simulink model "DSR_sim"  (R2021a)
settings: Solver=VariableStepAuto  StartTime=0.0  StopTime=15  RelTol=1e-3
undefined symbols (not defined in the file or in its folder): a, alpha, betac, delay, delay_a, omega
(part 1 of 2)
settings Model: Creator=shiva  LastModifiedBy=shiva

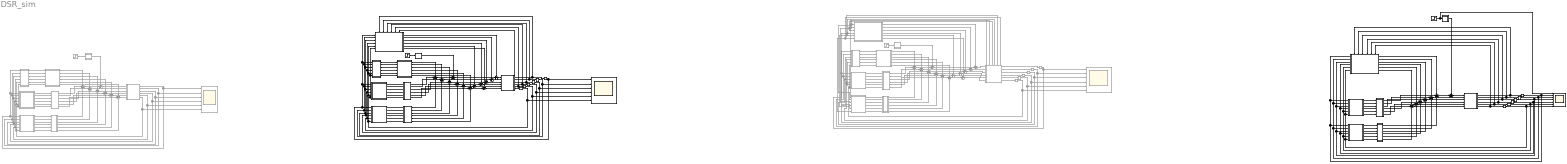
== system DSR_sim ==
  note: Standard Consensus
  note: DSR with velocity derivative
  note: System with accessible velocities
  ConsSys : Subsystem
  Damping : Subsystem
      settings: PortSchema="{\"entries\":[{\"content\":{\"sides\":[{\"content\":{\"connectorIds\":[\"In1\",\"In2\",\"In3\",\"In4\",\"In5\",\"In6\"]},\"type\":\"ConnectorPlacement.EquallySpacedRectSide\",\"uuid\":\"b372a7be-6970-4f0c-9c0a-91cfb5e8dee7\"},{\"content\":{\"connectorIds\":[\"Out1\",\"Out2\",\"Out3\",\"Out4\",\"Out5\",\"Out6\"],\"side\":\"RIGHT\"},\"type\":\"ConnectorPlacement.EquallySpacedRectSide\",\"uuid\":\"0b2444b3-7469-468f-9337-a7c17c408c74\"},{\"content\":{\"connectorIds\":[\"In7\",\"In8\",\"In9\",\"In10\",\"In11\",\"In12\"],\"side\":\"TOP\"},\"type\":\"ConnectorPlacement.EquallySpacedRectSide\",\"uuid\":\"794abe9b-397a-493b-b826-dc3a29ebdba9\"}]},\"type\":\"ConnectorPlacement.EquallySpacedConnector\",\"uuid\":\"dc72dcb4-42f7-41e7-aada-30e307c7b164\"}],\"packageUris\":[\"http://schema.mathworks.com/mf0/Connector/R2020b\"],\"version\":\"1.0\"}"
  Damping1 : Subsystem  Commented=on
  Damping2 : Subsystem
      settings: PortSchema="{\"entries\":[{\"content\":{\"sides\":[{\"content\":{\"connectorIds\":[\"In1\",\"In2\",\"In3\",\"In4\",\"In5\",\"In6\"]},\"type\":\"ConnectorPlacement.EquallySpacedRectSide\",\"uuid\":\"b372a7be-6970-4f0c-9c0a-91cfb5e8dee7\"},{\"content\":{\"connectorIds\":[\"Out1\",\"Out2\",\"Out3\",\"Out4\",\"Out5\",\"Out6\"],\"side\":\"RIGHT\"},\"type\":\"ConnectorPlacement.EquallySpacedRectSide\",\"uuid\":\"0b2444b3-7469-468f-9337-a7c17c408c74\"},{\"content\":{\"connectorIds\":[\"In7\",\"In8\",\"In9\",\"In10\",\"In11\",\"In12\"],\"side\":\"TOP\"},\"type\":\"ConnectorPlacement.EquallySpacedRectSide\",\"uuid\":\"794abe9b-397a-493b-b826-dc3a29ebdba9\"}]},\"type\":\"ConnectorPlacement.EquallySpacedConnector\",\"uuid\":\"dc72dcb4-42f7-41e7-aada-30e307c7b164\"}],\"packageUris\":[\"http://schema.mathworks.com/mf0/Connector/R2020b\"],\"version\":\"1.0\"}"
  DerEst : Subsystem  Commented=on
  DerEst1 : Subsystem
  DerEst2 : Subsystem  Commented=on
  I-beta*K : Subsystem  Commented=on
  I-beta*K1 : Subsystem
  I-beta*K2 : Subsystem  Commented=on
  Input Processor : Subsystem  Commented=on
  Input Processor1 : Subsystem
  Input Processor2 : Subsystem  Commented=on
  Input Processor3 : Subsystem
  KDgain : Subsystem  Commented=on
  KDgain1 : Subsystem
  KDgain2 : Subsystem  Commented=on
  KDgain3 : Subsystem
  KPgain : Subsystem  Commented=on
  KPgain1 : Subsystem
  KPgain2 : Subsystem  Commented=on
  KPgain3 : Subsystem
  KX : Subsystem  Commented=on
  KX1 : Subsystem
  KX2 : Subsystem  Commented=on
  KX3 : Subsystem
  KX_dot : Subsystem  Commented=on
  KX_dot1 : Subsystem
  KX_dot2 : Subsystem  Commented=on
  KX_dot3 : Subsystem
  Scope : Scope  Commented=on  NumInputPorts=6
  Scope1 : Scope  NumInputPorts=6
  Scope2 : Scope  Commented=on  NumInputPorts=6
  Scope4 : Scope  NumInputPorts=7
  Step : Step  Commented=on  SampleTime=0
  Step1 : Step  Time=0  SampleTime=0
  Step2 : Step  Commented=on  Time=0  SampleTime=0
  Step4 : Step  Time=0  SampleTime=0
  Sum{,1..5,20..22,30..32} (12 alike) : Sum  Commented=on  Inputs=+--
  Sum{7..12} (6 alike) : Sum  Inputs=+--
  Sum13 : Sum  Inputs=++|
  Sum{14..19} (6 alike) : Sum  Inputs=-+|
  Sum23 : Sum  Commented=on  Inputs=++|
  Sum{24..29} (6 alike) : Sum  Commented=on  Inputs=-+|
  Sum44 : Sum  Inputs=++|
  Sum{45..50} (6 alike) : Sum  Inputs=---
  Sum6 : Sum  Commented=on  Inputs=++|
  Transport Delay{,1..5,12..17} (12 alike) : TransportDelay  DelayTime=delay_a
  Transport Delay{6..11} (6 alike) : TransportDelay  Commented=on  DelayTime=delay_a
  system : Subsystem  Commented=on
  system1 : Subsystem
  system2 : Subsystem  Commented=on
      settings: PortSchema="{\"entries\":[{\"content\":{\"sides\":[{\"content\":{\"connectorIds\":[\"In1\",\"In2\",\"In3\",\"In4\",\"In5\",\"In6\"]},\"type\":\"ConnectorPlacement.EquallySpacedRectSide\",\"uuid\":\"0544da1f-0f67-4d19-801a-c3e0761d5fdd\"},{\"content\":{\"connectorIds\":[\"Out1\",\"Out2\",\"Out3\",\"Out4\",\"Out5\",\"Out6\"],\"side\":\"RIGHT\"},\"type\":\"ConnectorPlacement.EquallySpacedRectSide\",\"uuid\":\"07850a4a-c00e-49e5-b307-7878de70a2bd\"},{\"content\":{\"connectorIds\":[\"Out7\",\"Out8\",\"Out9\",\"Out10\",\"Out11\",\"Out12\"],\"side\":\"TOP\"},\"type\":\"ConnectorPlacement.EquallySpacedRectSide\",\"uuid\":\"1abf911a-7163-4aef-a115-7988dbad9a54\"}]},\"type\":\"ConnectorPlacement.EquallySpacedConnector\",\"uuid\":\"835a7fab-0379-4bf8-b1b3-ead7ebcc18b2\"}],\"packageUris\":[\"http://schema.mathworks.com/mf0/Connector/R2020b\"],\"version\":\"1.0\"}"
  wires:
  DerEst/1(est) -> I-beta*K/1(Input)
  DerEst/2(est1) -> I-beta*K/2(Input1)
  DerEst/3(est2) -> I-beta*K/3(Input2)
  DerEst/4(est3) -> I-beta*K/4(Input3)
  DerEst/5(est4) -> I-beta*K/5(Input4)
  DerEst/6(est5) -> I-beta*K/6(Input5)
  KX/1(Output) -> KPgain/1(Output)
  KX/2(Output1) -> KPgain/2(Output1)
  KX/3(Output2) -> KPgain/3(Output2)
  KX/4(Output3) -> KPgain/4(Output3)
  KX/5(Output4) -> KPgain/5(Output4)
  KX/6(Output5) -> KPgain/6(Output5)
  KX_dot/1(Output) -> KDgain/1(Output)
  KX_dot/2(Output1) -> KDgain/2(Output1)
  KX_dot/3(Output2) -> KDgain/3(Output2)
  KX_dot/4(Output3) -> KDgain/4(Output3)
  KX_dot/5(Output4) -> KDgain/5(Output4)
  KX_dot/6(Output5) -> KDgain/6(Output5)
  system/1(Ag1) -> KX_dot/1(Input), KX/1(Input), DerEst/1(pos), Scope/1
  system/2(Ag2) -> KX_dot/2(Input1), KX/2(Input1), DerEst/2(pos1), Scope/2
  system/3(Ag3) -> KX_dot/3(Input2), KX/3(Input2), DerEst/3(pos2), Scope/3
  system/4(Ag4) -> KX_dot/4(Input3), KX/4(Input3), DerEst/4(pos3), Scope/4
  system/5(Ag5) -> KX_dot/5(Input4), KX/5(Input4), DerEst/5(pos4), Scope/5
  system/6(Ag6) -> DerEst/6(pos5), KX/6(Input5), KX_dot/6(Input5), Scope/6
  Sum1/1 -> system/2(In2)
  Sum5/1 -> system/6(In6)
  Sum4/1 -> system/5(In5)
  Sum3/1 -> system/4(In4)
  Sum2/1 -> system/3(In3)
  Step/1 -> Input Processor/1(Input)
  Sum/1 -> Sum6/2
  Sum6/1 -> system/1(In1)
  Input Processor/1(Out1) -> Sum6/1
  I-beta*K/1(Output) -> Sum/1
  KPgain/1(Out1) -> Sum/2
  KDgain/1(Out1) -> Sum/3
  I-beta*K/2(Output1) -> Sum1/1
  KPgain/2(Out2) -> Sum1/2
  KDgain/2(Out2) -> Sum1/3
  I-beta*K/3(Output2) -> Sum2/1
  KPgain/3(Out3) -> Sum2/2
  KDgain/3(Out3) -> Sum2/3
  I-beta*K/4(Output3) -> Sum3/1
  KPgain/4(Out4) -> Sum3/2
  KDgain/4(Out4) -> Sum3/3
  I-beta*K/5(Output4) -> Sum4/1
  KPgain/5(Out5) -> Sum4/2
  KDgain/5(Out5) -> Sum4/3
  I-beta*K/6(Output5) -> Sum5/1
  KPgain/6(Out6) -> Sum5/2
  KDgain/6(Out6) -> Sum5/3
  KX1/4(Output3) -> KPgain1/4(Output3)
  KX1/6(Output5) -> KPgain1/6(Output5)
  KX1/2(Output1) -> KPgain1/2(Output1)
  I-beta*K1/1(Output) -> Sum7/1
  KX_dot1/3(Output2) -> KDgain1/3(Output2)
  I-beta*K1/6(Output5) -> Sum12/1
  system1/5(Ag5) -> Damping/11(Input7), Transport Delay4/1
  system1/4(Ag4) -> Transport Delay3/1, Damping/10(Input8)
  KPgain1/4(Out4) -> Sum10/2
  system1/2(Ag2) -> Transport Delay1/1, Damping/8(Input10)
  I-beta*K1/5(Output4) -> Sum11/1
  KPgain1/3(Out3) -> Sum9/2
  KX1/1(Output) -> KPgain1/1(Output)
  KX_dot1/5(Output4) -> KDgain1/5(Output4)
  system1/3(Ag3) -> Transport Delay2/1, Damping/9(Input9)
  KX_dot1/2(Output1) -> KDgain1/2(Output1)
  KX_dot1/6(Output5) -> KDgain1/6(Output5)
  Step1/1 -> Input Processor1/1(Input)
  KDgain1/4(Out4) -> Sum10/3
  KX1/5(Output4) -> KPgain1/5(Output4)
  KX_dot1/1(Output) -> KDgain1/1(Output)
  I-beta*K1/3(Output2) -> Sum9/1
  KPgain1/1(Out1) -> Sum7/2
  KDgain1/1(Out1) -> Sum7/3
  KDgain1/5(Out5) -> Sum11/3
  system1/6(Ag6) -> Transport Delay5/1, Damping/12(Input6)
  DerEst1/5(est4) -> I-beta*K1/5(Input4)
  system1/1(Ag1) -> Transport Delay/1, Damping/7(Input11)
  KPgain1/6(Out6) -> Sum12/2
  Sum7/1 -> Sum13/2
  I-beta*K1/4(Output3) -> Sum10/1
  KDgain1/3(Out3) -> Sum9/3
  KX1/3(Output2) -> KPgain1/3(Output2)
  Input Processor1/1(Out1) -> Sum13/1
  DerEst1/6(est5) -> I-beta*K1/6(Input5)
  KX_dot1/4(Output3) -> KDgain1/4(Output3)
  DerEst1/2(est1) -> I-beta*K1/2(Input1)
  KPgain1/5(Out5) -> Sum11/2
  KPgain1/2(Out2) -> Sum8/2
  KDgain1/2(Out2) -> Sum8/3
  DerEst1/4(est3) -> I-beta*K1/4(Input3)
  DerEst1/1(est) -> I-beta*K1/1(Input)
  KDgain1/6(Out6) -> Sum12/3
  DerEst1/3(est2) -> I-beta*K1/3(Input2)
  I-beta*K1/2(Output1) -> Sum8/1
  Sum14/1 -> system1/1(In1)
  Sum15/1 -> system1/2(In2)
  Sum16/1 -> system1/3(In3)
  Sum17/1 -> system1/4(In4)
  Sum18/1 -> system1/5(In5)
  Sum19/1 -> system1/6(In6)
  Sum12/1 -> Sum19/2
  Sum11/1 -> Sum18/2
  Sum10/1 -> Sum17/2
  Sum9/1 -> Sum16/2
  Sum8/1 -> Sum15/2
  Sum13/1 -> Sum14/2
  Transport Delay/1 -> KX_dot1/1(Input), KX1/1(Input), DerEst1/1(pos), Damping/1(Input), Scope1/1
  Transport Delay1/1 -> KX_dot1/2(Input1), KX1/2(Input1), DerEst1/2(pos1), Damping/2(Input1), Scope1/2
  Transport Delay2/1 -> KX_dot1/3(Input2), KX1/3(Input2), DerEst1/3(pos2), Damping/3(Input2), Scope1/3
  Transport Delay3/1 -> KX_dot1/4(Input3), KX1/4(Input3), DerEst1/4(pos3), Damping/4(Input3), Scope1/4
  Transport Delay4/1 -> KX_dot1/5(Input4), KX1/5(Input4), DerEst1/5(pos4), Damping/5(Input4), Scope1/5
  Transport Delay5/1 -> Damping/6(Input5), DerEst1/6(pos5), KX1/6(Input5), KX_dot1/6(Input5), Scope1/6
  Damping/1(Out1) -> Sum14/1
  Damping/2(Out2) -> Sum15/1
  Damping/3(Out3) -> Sum16/1
  Damping/4(Out4) -> Sum17/1
  Damping/5(Out5) -> Sum18/1
  Damping/6(Out6) -> Sum19/1
  Damping1/2(Out2) -> Sum25/1
  Damping1/1(Out1) -> Sum24/1
  Damping1/4(Out4) -> Sum27/1
  Damping1/5(Out5) -> Sum28/1
  Transport Delay11/1 -> DerEst2/6(pos5), KX2/6(Input5), Scope2/6
  Sum31/1 -> Sum25/2
  Sum23/1 -> Sum24/2
  Sum22/1 -> Sum29/2
  Sum26/1 -> system2/3(In3)
  Transport Delay10/1 -> KX2/5(Input4), DerEst2/5(pos4), Scope2/5
  Sum28/1 -> system2/5(In5)
  Sum27/1 -> system2/4(In4)
  Sum29/1 -> system2/6(In6)
  Sum20/1 -> Sum27/2
  Sum25/1 -> system2/2(In2)
  KDgain2/5(Out5) -> Sum21/3
  KDgain2/1(Out1) -> Sum30/3
  KPgain2/1(Out1) -> Sum30/2
  KDgain2/4(Out4) -> Sum20/3
  Step2/1 -> Input Processor2/1(Input)
  KX_dot2/1(Output) -> KDgain2/1(Output)
  KX_dot2/6(Output5) -> KDgain2/6(Output5)
  I-beta*K2/3(Output2) -> Sum32/1
  KX2/5(Output4) -> KPgain2/5(Output4)
  system2/3(Ag3) -> Transport Delay8/1
  KX_dot2/2(Output1) -> KDgain2/2(Output1)
  KPgain2/3(Out3) -> Sum32/2
  KX2/1(Output) -> KPgain2/1(Output)
  KX_dot2/5(Output4) -> KDgain2/5(Output4)
  I-beta*K2/5(Output4) -> Sum21/1
  system2/2(Ag2) -> Transport Delay7/1
  KPgain2/4(Out4) -> Sum20/2
  I-beta*K2/6(Output5) -> Sum22/1
  KX2/2(Output1) -> KPgain2/2(Output1)
  KX2/6(Output5) -> KPgain2/6(Output5)
  KPgain2/2(Out2) -> Sum31/2
  KDgain2/2(Out2) -> Sum31/3
  system2/5(Ag5) -> Transport Delay10/1
  DerEst2/1(est) -> I-beta*K2/1(Input)
  DerEst2/2(est1) -> I-beta*K2/2(Input1)
  system2/4(Ag4) -> Transport Delay9/1
  Input Processor2/1(Out1) -> Sum23/1
  KX_dot2/4(Output3) -> KDgain2/4(Output3)
  KX2/3(Output2) -> KPgain2/3(Output2)
  DerEst2/6(est5) -> I-beta*K2/6(Input5)
  Sum32/1 -> Sum26/2
  I-beta*K2/4(Output3) -> Sum20/1
  Sum30/1 -> Sum23/2
  KDgain2/6(Out6) -> Sum22/3
  DerEst2/4(est3) -> I-beta*K2/4(Input3)
  KX_dot2/3(Output2) -> KDgain2/3(Output2)
  KDgain2/3(Out3) -> Sum32/3
  system2/1(Ag1) -> Transport Delay6/1
  KPgain2/6(Out6) -> Sum22/2
  Sum21/1 -> Sum28/2
  DerEst2/5(est4) -> I-beta*K2/5(Input4)
  DerEst2/3(est2) -> I-beta*K2/3(Input2)
  system2/6(Ag6) -> Transport Delay11/1
  Transport Delay9/1 -> KX2/4(Input3), DerEst2/4(pos3), Scope2/4
  Damping1/6(Out6) -> Sum29/1
  Transport Delay6/1 -> KX2/1(Input), DerEst2/1(pos), Scope2/1
  KX2/4(Output3) -> KPgain2/4(Output3)
  I-beta*K2/1(Output) -> Sum30/1
  Transport Delay8/1 -> KX2/3(Input2), DerEst2/3(pos2), Scope2/3
  Transport Delay7/1 -> KX2/2(Input1), DerEst2/2(pos1), Scope2/2
  I-beta*K2/2(Output1) -> Sum31/1
  KPgain2/5(Out5) -> Sum21/2
  Sum24/1 -> system2/1(In1)
  Damping1/3(Out3) -> Sum26/1
  system2/7(Ag7) -> KX_dot2/1(Input), Damping1/1(Input)
  system2/8(Ag8) -> KX_dot2/2(Input1), Damping1/2(Input1)
  system2/9(Ag9) -> KX_dot2/3(Input2), Damping1/3(Input2)
  system2/10(Ag10) -> Damping1/4(Input3), KX_dot2/4(Input3)
  system2/11(Ag11) -> KX_dot2/5(Input4), Damping1/5(Input4)
  system2/12(Ag12) -> Damping1/6(Input5), KX_dot2/6(Input5)
  ConsSys/6(Ag6) -> Damping2/12(Input6), Transport Delay17/1
  ConsSys/5(Ag5) -> Damping2/11(Input7), Transport Delay16/1
  ConsSys/4(Ag4) -> Damping2/10(Input8), Transport Delay15/1
  ConsSys/3(Ag3) -> Damping2/9(Input9), Transport Delay14/1
  ConsSys/2(Ag2) -> Transport Delay13/1, Damping2/8(Input10)
  ConsSys/1(Ag1) -> Damping2/7(Input11), Transport Delay12/1
  KX3/1(Output) -> KPgain3/1(Output)
  KX3/2(Output1) -> KPgain3/2(Output1)
  KX3/3(Output2) -> KPgain3/3(Output2)
  KX3/4(Output3) -> KPgain3/4(Output3)
  KX3/5(Output4) -> KPgain3/5(Output4)
  KX3/6(Output5) -> KPgain3/6(Output5)
  Step4/1 -> Scope4/1, Input Processor3/1(Input)
  KX_dot3/1(Output) -> KDgain3/1(Output)
  KX_dot3/2(Output1) -> KDgain3/2(Output1)
  KX_dot3/3(Output2) -> KDgain3/3(Output2)
  KX_dot3/4(Output3) -> KDgain3/4(Output3)
  KX_dot3/5(Output4) -> KDgain3/5(Output4)
  KX_dot3/6(Output5) -> KDgain3/6(Output5)
  Transport Delay12/1 -> Damping2/1(Input), KX3/1(Input), KX_dot3/1(Input), Scope4/2
  Transport Delay13/1 -> Damping2/2(Input1), KX3/2(Input1), KX_dot3/2(Input1), Scope4/3
  Transport Delay14/1 -> Damping2/3(Input2), KX3/3(Input2), KX_dot3/3(Input2), Scope4/4
  Transport Delay15/1 -> Damping2/4(Input3), KX3/4(Input3), KX_dot3/4(Input3), Scope4/5
  Transport Delay16/1 -> Damping2/5(Input4), KX3/5(Input4), KX_dot3/5(Input4), Scope4/6
  Transport Delay17/1 -> Damping2/6(Input5), KX3/6(Input5), KX_dot3/6(Input5), Scope4/7
  Sum46/1 -> ConsSys/2(In2)
  Sum44/1 -> ConsSys/1(In1)
  Sum45/1 -> Sum44/2
  Sum48/1 -> ConsSys/4(In4)
  Sum49/1 -> ConsSys/5(In5)
  Sum50/1 -> ConsSys/6(In6)
  Sum47/1 -> ConsSys/3(In3)
  Input Processor3/1(Out1) -> Sum44/1
  KPgain3/1(Out1) -> Sum45/2
  KPgain3/2(Out2) -> Sum46/2
  KPgain3/3(Out3) -> Sum47/2
  KPgain3/4(Out4) -> Sum48/2
  KPgain3/5(Out5) -> Sum49/2
  KPgain3/6(Out6) -> Sum50/2
  KDgain3/1(Out1) -> Sum45/3
  KDgain3/2(Out2) -> Sum46/3
  KDgain3/3(Out3) -> Sum47/3
  KDgain3/4(Out4) -> Sum48/3
  KDgain3/5(Out5) -> Sum49/3
  KDgain3/6(Out6) -> Sum50/3
  Damping2/1(Out1) -> Sum45/1
  Damping2/2(Out2) -> Sum46/1
  Damping2/3(Out3) -> Sum47/1
  Damping2/4(Out4) -> Sum48/1
  Damping2/5(Out5) -> Sum49/1
  Damping2/6(Out6) -> Sum50/1

== system DSR_sim/ConsSys ==
  In1 : Inport
  In2 : Inport  Port=2
  In3 : Inport  Port=3
  In4 : Inport  Port=4
  In5 : Inport  Port=5
  In6 : Inport  Port=6
  Transfer Fcn{,1..5} (6 alike) : TransferFcn  Denominator=[1 0 0]
  Ag1 : Outport
  Ag2 : Outport  Port=2
  Ag3 : Outport  Port=3
  Ag4 : Outport  Port=4
  Ag5 : Outport  Port=5
  Ag6 : Outport  Port=6
  wires:
  Transfer Fcn4/1 -> Ag5/1
  In1/1 -> Transfer Fcn/1
  Transfer Fcn/1 -> Ag1/1
  In3/1 -> Transfer Fcn2/1
  Transfer Fcn2/1 -> Ag3/1
  In2/1 -> Transfer Fcn1/1
  In5/1 -> Transfer Fcn4/1
  Transfer Fcn1/1 -> Ag2/1
  In6/1 -> Transfer Fcn5/1
  In4/1 -> Transfer Fcn3/1
  Transfer Fcn5/1 -> Ag6/1
  Transfer Fcn3/1 -> Ag4/1

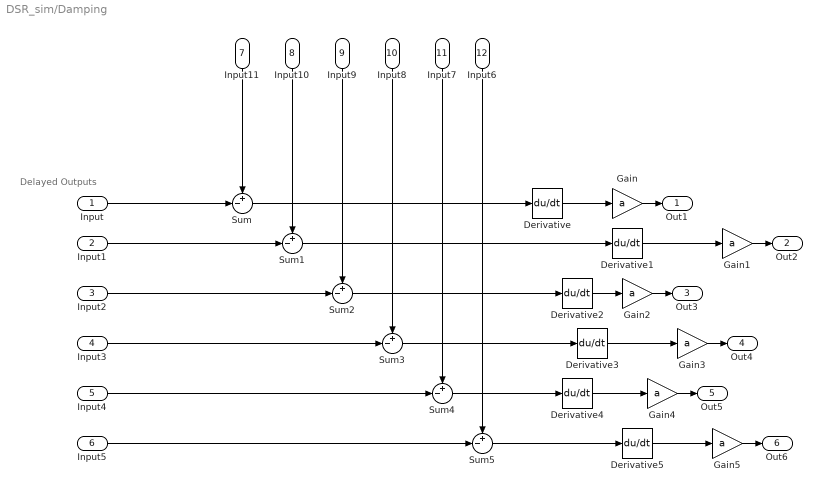
== system DSR_sim/Damping ==
  note: Delayed Outputs
  Input : Inport
  Input1 : Inport  Port=2
  Input2 : Inport  Port=3
  Input3 : Inport  Port=4
  Input4 : Inport  Port=5
  Input5 : Inport  Port=6
  Input11 : Inport  Port=7
  Input10 : Inport  Port=8
  Input9 : Inport  Port=9
  Input8 : Inport  Port=10
  Input7 : Inport  Port=11
  Input6 : Inport  Port=12
  Derivative{,1..5} (6 alike) : Derivative
  Gain{,1..5} (6 alike) : Gain  Gain=a
  Sum{,1..5} (6 alike) : Sum  Inputs=+-|
  Out1 : Outport
  Out2 : Outport  Port=2
  Out3 : Outport  Port=3
  Out4 : Outport  Port=4
  Out5 : Outport  Port=5
  Out6 : Outport  Port=6
  wires:
  Gain5/1 -> Out6/1
  Gain/1 -> Out1/1
  Gain2/1 -> Out3/1
  Gain4/1 -> Out5/1
  Gain3/1 -> Out4/1
  Gain1/1 -> Out2/1
  Input/1 -> Sum/2
  Input11/1 -> Sum/1
  Sum/1 -> Derivative/1
  Input1/1 -> Sum1/2
  Input10/1 -> Sum1/1
  Input2/1 -> Sum2/2
  Input9/1 -> Sum2/1
  Input8/1 -> Sum3/1
  Input3/1 -> Sum3/2
  Input4/1 -> Sum4/2
  Input7/1 -> Sum4/1
  Input5/1 -> Sum5/2
  Input6/1 -> Sum5/1
  Sum1/1 -> Derivative1/1
  Sum2/1 -> Derivative2/1
  Sum3/1 -> Derivative3/1
  Sum4/1 -> Derivative4/1
  Sum5/1 -> Derivative5/1
  Derivative/1 -> Gain/1
  Derivative1/1 -> Gain1/1
  Derivative2/1 -> Gain2/1
  Derivative3/1 -> Gain3/1
  Derivative4/1 -> Gain4/1
  Derivative5/1 -> Gain5/1

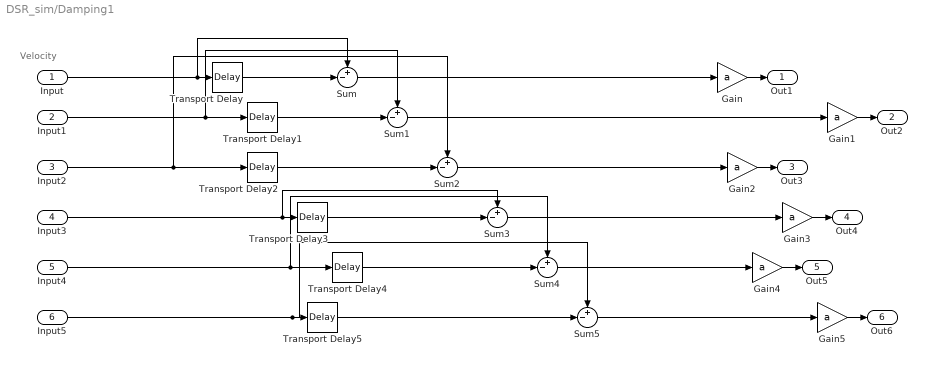
== system DSR_sim/Damping1 ==
  note: Velocity
  Input : Inport
  Input1 : Inport  Port=2
  Input2 : Inport  Port=3
  Input3 : Inport  Port=4
  Input4 : Inport  Port=5
  Input5 : Inport  Port=6
  Gain{,1..5} (6 alike) : Gain  Gain=a
  Sum{,1..5} (6 alike) : Sum  Inputs=+-|
  Transport Delay{,1..5} (6 alike) : TransportDelay  DelayTime=delay_a
  Out1 : Outport
  Out2 : Outport  Port=2
  Out3 : Outport  Port=3
  Out4 : Outport  Port=4
  Out5 : Outport  Port=5
  Out6 : Outport  Port=6
  wires:
  Gain5/1 -> Out6/1
  Gain/1 -> Out1/1
  Gain2/1 -> Out3/1
  Gain4/1 -> Out5/1
  Gain3/1 -> Out4/1
  Gain1/1 -> Out2/1
  Input/1 -> Sum/1, Transport Delay/1
  Input1/1 -> Transport Delay1/1, Sum1/1
  Input2/1 -> Transport Delay2/1, Sum2/1
  Input3/1 -> Sum3/1, Transport Delay3/1
  Input4/1 -> Transport Delay4/1, Sum4/1
  Input5/1 -> Sum5/1, Transport Delay5/1
  Sum/1 -> Gain/1
  Sum1/1 -> Gain1/1
  Sum2/1 -> Gain2/1
  Sum3/1 -> Gain3/1
  Sum4/1 -> Gain4/1
  Sum5/1 -> Gain5/1
  Transport Delay/1 -> Sum/2
  Transport Delay1/1 -> Sum1/2
  Transport Delay2/1 -> Sum2/2
  Transport Delay3/1 -> Sum3/2
  Transport Delay4/1 -> Sum4/2
  Transport Delay5/1 -> Sum5/2

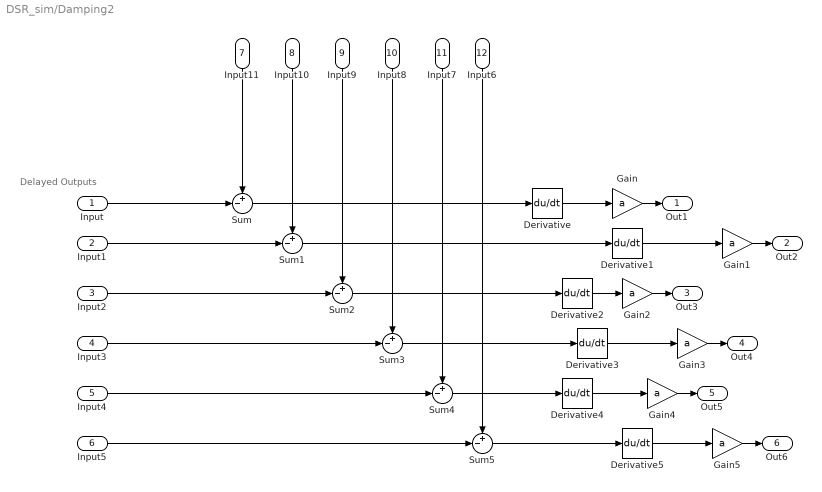
== system DSR_sim/Damping2 ==
  note: Delayed Outputs
  Input : Inport
  Input1 : Inport  Port=2
  Input2 : Inport  Port=3
  Input3 : Inport  Port=4
  Input4 : Inport  Port=5
  Input5 : Inport  Port=6
  Input11 : Inport  Port=7
  Input10 : Inport  Port=8
  Input9 : Inport  Port=9
  Input8 : Inport  Port=10
  Input7 : Inport  Port=11
  Input6 : Inport  Port=12
  Derivative{,1..5} (6 alike) : Derivative
  Gain{,1..5} (6 alike) : Gain  Gain=a
  Sum{,1..5} (6 alike) : Sum  Inputs=+-|
  Out1 : Outport
  Out2 : Outport  Port=2
  Out3 : Outport  Port=3
  Out4 : Outport  Port=4
  Out5 : Outport  Port=5
  Out6 : Outport  Port=6
  wires:
  Gain5/1 -> Out6/1
  Gain/1 -> Out1/1
  Gain2/1 -> Out3/1
  Gain4/1 -> Out5/1
  Gain3/1 -> Out4/1
  Gain1/1 -> Out2/1
  Input/1 -> Sum/2
  Input11/1 -> Sum/1
  Sum/1 -> Derivative/1
  Input1/1 -> Sum1/2
  Input10/1 -> Sum1/1
  Input2/1 -> Sum2/2
  Input9/1 -> Sum2/1
  Input8/1 -> Sum3/1
  Input3/1 -> Sum3/2
  Input4/1 -> Sum4/2
  Input7/1 -> Sum4/1
  Input5/1 -> Sum5/2
  Input6/1 -> Sum5/1
  Sum1/1 -> Derivative1/1
  Sum2/1 -> Derivative2/1
  Sum3/1 -> Derivative3/1
  Sum4/1 -> Derivative4/1
  Sum5/1 -> Derivative5/1
  Derivative/1 -> Gain/1
  Derivative1/1 -> Gain1/1
  Derivative2/1 -> Gain2/1
  Derivative3/1 -> Gain3/1
  Derivative4/1 -> Gain4/1
  Derivative5/1 -> Gain5/1

== system DSR_sim/DerEst ==
  pos : Inport
  pos1 : Inport  Port=2
  pos2 : Inport  Port=3
  pos3 : Inport  Port=4
  pos4 : Inport  Port=5
  pos5 : Inport  Port=6
  Derivative Estimator : Subsystem
  Derivative Estimator1 : Subsystem
  Derivative Estimator2 : Subsystem
  Derivative Estimator3 : Subsystem
  Derivative Estimator4 : Subsystem
  Derivative Estimator5 : Subsystem
  est : Outport
  est1 : Outport  Port=2
  est2 : Outport  Port=3
  est3 : Outport  Port=4
  est4 : Outport  Port=5
  est5 : Outport  Port=6
  wires:
  pos3/1 -> Derivative Estimator3/1(pos)
  Derivative Estimator4/1(est) -> est4/1
  Derivative Estimator2/1(est) -> est2/1
  Derivative Estimator3/1(est) -> est3/1
  Derivative Estimator1/1(est) -> est1/1
  pos1/1 -> Derivative Estimator1/1(pos)
  Derivative Estimator5/1(est) -> est5/1
  Derivative Estimator/1(est) -> est/1
  pos/1 -> Derivative Estimator/1(pos)
  pos2/1 -> Derivative Estimator2/1(pos)
  pos5/1 -> Derivative Estimator5/1(pos)
  pos4/1 -> Derivative Estimator4/1(pos)

== system DSR_sim/DerEst1 ==
  pos : Inport
  pos1 : Inport  Port=2
  pos2 : Inport  Port=3
  pos3 : Inport  Port=4
  pos4 : Inport  Port=5
  pos5 : Inport  Port=6
  Derivative Estimator : Subsystem
  Derivative Estimator1 : Subsystem
  Derivative Estimator2 : Subsystem
  Derivative Estimator3 : Subsystem
  Derivative Estimator4 : Subsystem
  Derivative Estimator5 : Subsystem
  est : Outport
  est1 : Outport  Port=2
  est2 : Outport  Port=3
  est3 : Outport  Port=4
  est4 : Outport  Port=5
  est5 : Outport  Port=6
  wires:
  pos3/1 -> Derivative Estimator3/1(pos)
  Derivative Estimator4/1(est) -> est4/1
  Derivative Estimator2/1(est) -> est2/1
  Derivative Estimator3/1(est) -> est3/1
  Derivative Estimator1/1(est) -> est1/1
  pos1/1 -> Derivative Estimator1/1(pos)
  Derivative Estimator5/1(est) -> est5/1
  Derivative Estimator/1(est) -> est/1
  pos/1 -> Derivative Estimator/1(pos)
  pos2/1 -> Derivative Estimator2/1(pos)
  pos5/1 -> Derivative Estimator5/1(pos)
  pos4/1 -> Derivative Estimator4/1(pos)

== system DSR_sim/DerEst2 ==
  pos : Inport
  pos1 : Inport  Port=2
  pos2 : Inport  Port=3
  pos3 : Inport  Port=4
  pos4 : Inport  Port=5
  pos5 : Inport  Port=6
  Derivative Estimator : Subsystem
  Derivative Estimator1 : Subsystem
  Derivative Estimator2 : Subsystem
  Derivative Estimator3 : Subsystem
  Derivative Estimator4 : Subsystem
  Derivative Estimator5 : Subsystem
  est : Outport
  est1 : Outport  Port=2
  est2 : Outport  Port=3
  est3 : Outport  Port=4
  est4 : Outport  Port=5
  est5 : Outport  Port=6
  wires:
  pos3/1 -> Derivative Estimator3/1(pos)
  Derivative Estimator4/1(est) -> est4/1
  Derivative Estimator2/1(est) -> est2/1
  Derivative Estimator3/1(est) -> est3/1
  Derivative Estimator1/1(est) -> est1/1
  pos1/1 -> Derivative Estimator1/1(pos)
  Derivative Estimator5/1(est) -> est5/1
  Derivative Estimator/1(est) -> est/1
  pos/1 -> Derivative Estimator/1(pos)
  pos2/1 -> Derivative Estimator2/1(pos)
  pos5/1 -> Derivative Estimator5/1(pos)
  pos4/1 -> Derivative Estimator4/1(pos)

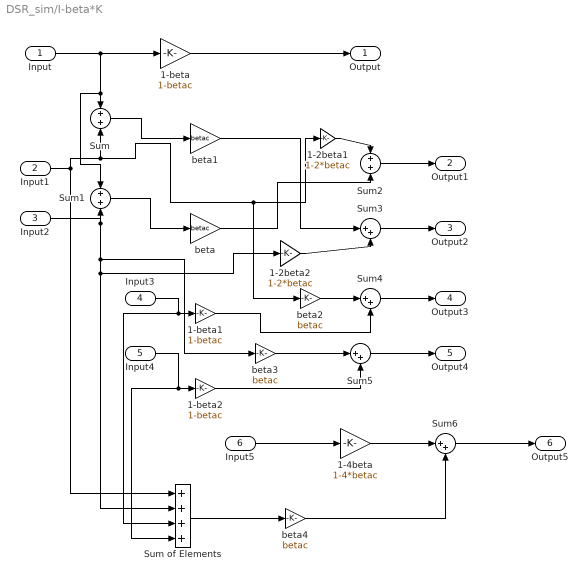
== system DSR_sim/I-beta*K ==
  Input : Inport
  Input1 : Inport  Port=2
  Input2 : Inport  Port=3
  Input3 : Inport  Port=4
  Input4 : Inport  Port=5
  Input5 : Inport  Port=6
  1-2beta1 : Gain  Gain=1-2*betac
  1-2beta2 : Gain  Gain=1-2*betac
  1-4beta : Gain  Gain=1-4*betac
  1-beta : Gain  Gain=1-betac
  1-beta1 : Gain  Gain=1-betac
  1-beta2 : Gain  Gain=1-betac
  Sum : Sum  Inputs=+|+
  Sum of Elements : Sum  Inputs=++++
  Sum1 : Sum  Inputs=+|+
  Sum2 : Sum  Inputs=+|+
  Sum{3..6} (4 alike) : Sum  Inputs=|++
  beta{,1..4} (5 alike) : Gain  Gain=betac
  Output : Outport
  Output1 : Outport  Port=2
  Output2 : Outport  Port=3
  Output3 : Outport  Port=4
  Output4 : Outport  Port=5
  Output5 : Outport  Port=6
  wires:
  Input/1 -> 1-beta/1, Sum1/1, Sum/1
  1-2beta2/1 -> Sum3/2
  1-beta2/1 -> Sum5/2
  Sum4/1 -> Output3/1
  1-beta/1 -> Output/1
  beta/1 -> Sum2/2
  Sum6/1 -> Output5/1
  1-beta1/1 -> Sum4/2
  Input2/1 -> Sum of Elements/2, 1-2beta2/1, beta3/1, Sum1/2
  1-2beta1/1 -> Sum2/1
  Input1/1 -> 1-2beta1/1, beta2/1, Sum/2, Sum of Elements/1
  beta4/1 -> Sum6/2
  Sum/1 -> beta1/1
  Input3/1 -> Sum of Elements/3, 1-beta1/1
  beta3/1 -> Sum5/1
  beta1/1 -> Sum3/1
  beta2/1 -> Sum4/1
  Sum5/1 -> Output4/1
  Input4/1 -> Sum of Elements/4, 1-beta2/1
  Sum1/1 -> beta/1
  1-4beta/1 -> Sum6/1
  Sum2/1 -> Output1/1
  Sum3/1 -> Output2/1
  Input5/1 -> 1-4beta/1
  Sum of Elements/1 -> beta4/1

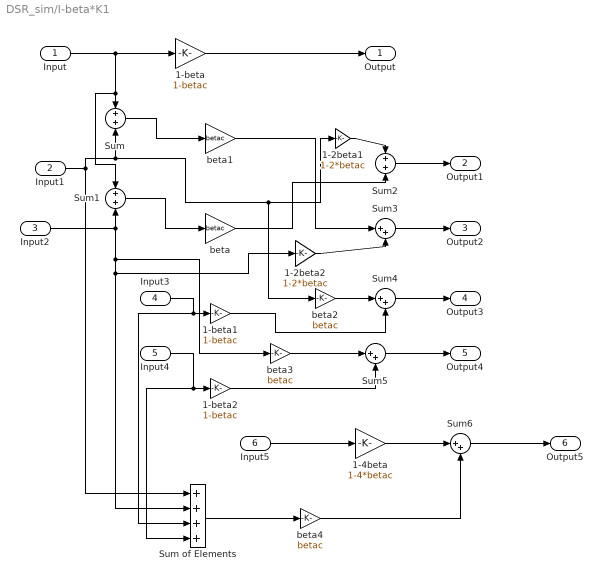
== system DSR_sim/I-beta*K1 ==
  Input : Inport
  Input1 : Inport  Port=2
  Input2 : Inport  Port=3
  Input3 : Inport  Port=4
  Input4 : Inport  Port=5
  Input5 : Inport  Port=6
  1-2beta1 : Gain  Gain=1-2*betac
  1-2beta2 : Gain  Gain=1-2*betac
  1-4beta : Gain  Gain=1-4*betac
  1-beta : Gain  Gain=1-betac
  1-beta1 : Gain  Gain=1-betac
  1-beta2 : Gain  Gain=1-betac
  Sum : Sum  Inputs=+|+
  Sum of Elements : Sum  Inputs=++++
  Sum1 : Sum  Inputs=+|+
  Sum2 : Sum  Inputs=+|+
  Sum{3..6} (4 alike) : Sum  Inputs=|++
  beta{,1..4} (5 alike) : Gain  Gain=betac
  Output : Outport
  Output1 : Outport  Port=2
  Output2 : Outport  Port=3
  Output3 : Outport  Port=4
  Output4 : Outport  Port=5
  Output5 : Outport  Port=6
  wires:
  Input/1 -> 1-beta/1, Sum1/1, Sum/1
  1-2beta2/1 -> Sum3/2
  1-beta2/1 -> Sum5/2
  Sum4/1 -> Output3/1
  1-beta/1 -> Output/1
  beta/1 -> Sum2/2
  Sum6/1 -> Output5/1
  1-beta1/1 -> Sum4/2
  Input2/1 -> Sum1/2, Sum of Elements/2, 1-2beta2/1, beta3/1
  1-2beta1/1 -> Sum2/1
  Input1/1 -> 1-2beta1/1, beta2/1, Sum/2, Sum of Elements/1
  beta4/1 -> Sum6/2
  Sum/1 -> beta1/1
  Input3/1 -> Sum of Elements/3, 1-beta1/1
  beta3/1 -> Sum5/1
  beta1/1 -> Sum3/1
  beta2/1 -> Sum4/1
  Sum5/1 -> Output4/1
  Input4/1 -> Sum of Elements/4, 1-beta2/1
  Sum1/1 -> beta/1
  1-4beta/1 -> Sum6/1
  Sum2/1 -> Output1/1
  Sum3/1 -> Output2/1
  Input5/1 -> 1-4beta/1
  Sum of Elements/1 -> beta4/1

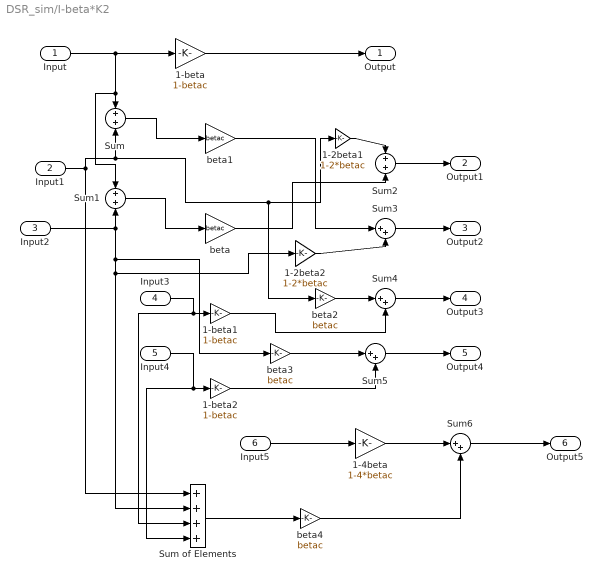
== system DSR_sim/I-beta*K2 ==
  Input : Inport
  Input1 : Inport  Port=2
  Input2 : Inport  Port=3
  Input3 : Inport  Port=4
  Input4 : Inport  Port=5
  Input5 : Inport  Port=6
  1-2beta1 : Gain  Gain=1-2*betac
  1-2beta2 : Gain  Gain=1-2*betac
  1-4beta : Gain  Gain=1-4*betac
  1-beta : Gain  Gain=1-betac
  1-beta1 : Gain  Gain=1-betac
  1-beta2 : Gain  Gain=1-betac
  Sum : Sum  Inputs=+|+
  Sum of Elements : Sum  Inputs=++++
  Sum1 : Sum  Inputs=+|+
  Sum2 : Sum  Inputs=+|+
  Sum{3..6} (4 alike) : Sum  Inputs=|++
  beta{,1..4} (5 alike) : Gain  Gain=betac
  Output : Outport
  Output1 : Outport  Port=2
  Output2 : Outport  Port=3
  Output3 : Outport  Port=4
  Output4 : Outport  Port=5
  Output5 : Outport  Port=6
  wires:
  Input/1 -> 1-beta/1, Sum1/1, Sum/1
  1-2beta2/1 -> Sum3/2
  1-beta2/1 -> Sum5/2
  Sum4/1 -> Output3/1
  1-beta/1 -> Output/1
  beta/1 -> Sum2/2
  Sum6/1 -> Output5/1
  1-beta1/1 -> Sum4/2
  Input2/1 -> Sum1/2, Sum of Elements/2, 1-2beta2/1, beta3/1
  1-2beta1/1 -> Sum2/1
  Input1/1 -> 1-2beta1/1, beta2/1, Sum/2, Sum of Elements/1
  beta4/1 -> Sum6/2
  Sum/1 -> beta1/1
  Input3/1 -> Sum of Elements/3, 1-beta1/1
  beta3/1 -> Sum5/1
  beta1/1 -> Sum3/1
  beta2/1 -> Sum4/1
  Sum5/1 -> Output4/1
  Input4/1 -> Sum of Elements/4, 1-beta2/1
  Sum1/1 -> beta/1
  1-4beta/1 -> Sum6/1
  Sum2/1 -> Output1/1
  Sum3/1 -> Output2/1
  Input5/1 -> 1-4beta/1
  Sum of Elements/1 -> beta4/1

== system DSR_sim/Input Processor ==
  Input : Inport
  Derivative : Derivative
  Gain : Gain  Gain=alpha
  Gain1 : Gain  Gain=2
  Sum : Sum  Inputs=|++
  inputGain : Gain  Gain=alpha*betac
  Out1 : Outport
  wires:
  Gain1/1 -> Sum/2
  Derivative/1 -> Gain1/1
  Input/1 -> Gain/1, Derivative/1
  Sum/1 -> inputGain/1
  Gain/1 -> Sum/1
  inputGain/1 -> Out1/1

== system DSR_sim/Input Processor1 ==
  Input : Inport
  Derivative : Derivative
  Gain : Gain  Gain=alpha
  Gain1 : Gain  Gain=2
  Sum : Sum  Inputs=|++
  inputGain : Gain  Gain=alpha*betac
  Out1 : Outport
  wires:
  Gain1/1 -> Sum/2
  Derivative/1 -> Gain1/1
  Input/1 -> Gain/1, Derivative/1
  Sum/1 -> inputGain/1
  Gain/1 -> Sum/1
  inputGain/1 -> Out1/1

== system DSR_sim/Input Processor2 ==
  Input : Inport
  Derivative : Derivative
  Gain : Gain  Gain=alpha
  Gain1 : Gain  Gain=2
  Sum : Sum  Inputs=|++
  inputGain : Gain  Gain=alpha*betac
  Out1 : Outport
  wires:
  Gain1/1 -> Sum/2
  Derivative/1 -> Gain1/1
  Input/1 -> Gain/1, Derivative/1
  Sum/1 -> inputGain/1
  Gain/1 -> Sum/1
  inputGain/1 -> Out1/1

== system DSR_sim/Input Processor3 ==
  Input : Inport
  Derivative : Derivative
  Gain : Gain  Gain=alpha
  Gain1 : Gain  Gain=2
  Sum : Sum  Inputs=|++
  inputGain : Gain  Gain=alpha
  Out1 : Outport
  wires:
  Gain1/1 -> Sum/2
  Derivative/1 -> Gain1/1
  Input/1 -> Gain/1, Derivative/1
  Sum/1 -> inputGain/1
  Gain/1 -> Sum/1
  inputGain/1 -> Out1/1

== system DSR_sim/KDgain ==
  Output : Inport
  Output1 : Inport  Port=2
  Output2 : Inport  Port=3
  Output3 : Inport  Port=4
  Output4 : Inport  Port=5
  Output5 : Inport  Port=6
  KDgain{2..7} (6 alike) : Gain  Gain=2*alpha*betac
  Out1 : Outport
  Out2 : Outport  Port=2
  Out3 : Outport  Port=3
  Out4 : Outport  Port=4
  Out5 : Outport  Port=5
  Out6 : Outport  Port=6
  wires:
  Output2/1 -> KDgain4/1
  KDgain4/1 -> Out3/1
  KDgain3/1 -> Out2/1
  KDgain6/1 -> Out5/1
  Output4/1 -> KDgain6/1
  Output/1 -> KDgain2/1
  KDgain2/1 -> Out1/1
  KDgain5/1 -> Out4/1
  Output3/1 -> KDgain5/1
  KDgain7/1 -> Out6/1
  Output5/1 -> KDgain7/1
  Output1/1 -> KDgain3/1

== system DSR_sim/KDgain1 ==
  Output : Inport
  Output1 : Inport  Port=2
  Output2 : Inport  Port=3
  Output3 : Inport  Port=4
  Output4 : Inport  Port=5
  Output5 : Inport  Port=6
  KDgain{2..7} (6 alike) : Gain  Gain=2*alpha*betac
  Out1 : Outport
  Out2 : Outport  Port=2
  Out3 : Outport  Port=3
  Out4 : Outport  Port=4
  Out5 : Outport  Port=5
  Out6 : Outport  Port=6
  wires:
  Output2/1 -> KDgain4/1
  KDgain4/1 -> Out3/1
  KDgain3/1 -> Out2/1
  KDgain6/1 -> Out5/1
  Output4/1 -> KDgain6/1
  Output/1 -> KDgain2/1
  KDgain2/1 -> Out1/1
  KDgain5/1 -> Out4/1
  Output3/1 -> KDgain5/1
  KDgain7/1 -> Out6/1
  Output5/1 -> KDgain7/1
  Output1/1 -> KDgain3/1

== system DSR_sim/KDgain2 ==
  Output : Inport
  Output1 : Inport  Port=2
  Output2 : Inport  Port=3
  Output3 : Inport  Port=4
  Output4 : Inport  Port=5
  Output5 : Inport  Port=6
  KDgain{2..7} (6 alike) : Gain  Gain=2*alpha*betac
  Out1 : Outport
  Out2 : Outport  Port=2
  Out3 : Outport  Port=3
  Out4 : Outport  Port=4
  Out5 : Outport  Port=5
  Out6 : Outport  Port=6
  wires:
  Output2/1 -> KDgain4/1
  KDgain4/1 -> Out3/1
  KDgain3/1 -> Out2/1
  KDgain6/1 -> Out5/1
  Output4/1 -> KDgain6/1
  Output/1 -> KDgain2/1
  KDgain2/1 -> Out1/1
  KDgain5/1 -> Out4/1
  Output3/1 -> KDgain5/1
  KDgain7/1 -> Out6/1
  Output5/1 -> KDgain7/1
  Output1/1 -> KDgain3/1

== system DSR_sim/KDgain3 ==
  Output : Inport
  Output1 : Inport  Port=2
  Output2 : Inport  Port=3
  Output3 : Inport  Port=4
  Output4 : Inport  Port=5
  Output5 : Inport  Port=6
  KDgain{2..7} (6 alike) : Gain  Gain=2*alpha
  Out1 : Outport
  Out2 : Outport  Port=2
  Out3 : Outport  Port=3
  Out4 : Outport  Port=4
  Out5 : Outport  Port=5
  Out6 : Outport  Port=6
  wires:
  Output2/1 -> KDgain4/1
  KDgain4/1 -> Out3/1
  KDgain3/1 -> Out2/1
  KDgain6/1 -> Out5/1
  Output4/1 -> KDgain6/1
  Output/1 -> KDgain2/1
  KDgain2/1 -> Out1/1
  KDgain5/1 -> Out4/1
  Output3/1 -> KDgain5/1
  KDgain7/1 -> Out6/1
  Output5/1 -> KDgain7/1
  Output1/1 -> KDgain3/1

== system DSR_sim/KPgain ==
  Output : Inport
  Output1 : Inport  Port=2
  Output2 : Inport  Port=3
  Output3 : Inport  Port=4
  Output4 : Inport  Port=5
  Output5 : Inport  Port=6
  KPgain{1..6} (6 alike) : Gain  Gain=alpha^2*betac
  Out1 : Outport
  Out2 : Outport  Port=2
  Out3 : Outport  Port=3
  Out4 : Outport  Port=4
  Out5 : Outport  Port=5
  Out6 : Outport  Port=6
  wires:
  Output4/1 -> KPgain5/1
  KPgain1/1 -> Out1/1
  KPgain2/1 -> Out2/1
  KPgain5/1 -> Out5/1
  Output/1 -> KPgain1/1
  Output3/1 -> KPgain4/1
  Output5/1 -> KPgain6/1
  Output1/1 -> KPgain2/1
  KPgain3/1 -> Out3/1
  KPgain6/1 -> Out6/1
  Output2/1 -> KPgain3/1
  KPgain4/1 -> Out4/1

== system DSR_sim/KPgain1 ==
  Output : Inport
  Output1 : Inport  Port=2
  Output2 : Inport  Port=3
  Output3 : Inport  Port=4
  Output4 : Inport  Port=5
  Output5 : Inport  Port=6
  KPgain{1..6} (6 alike) : Gain  Gain=betac*alpha^2
  Out1 : Outport
  Out2 : Outport  Port=2
  Out3 : Outport  Port=3
  Out4 : Outport  Port=4
  Out5 : Outport  Port=5
  Out6 : Outport  Port=6
  wires:
  Output4/1 -> KPgain5/1
  KPgain1/1 -> Out1/1
  KPgain2/1 -> Out2/1
  KPgain5/1 -> Out5/1
  Output/1 -> KPgain1/1
  Output3/1 -> KPgain4/1
  Output5/1 -> KPgain6/1
  Output1/1 -> KPgain2/1
  KPgain3/1 -> Out3/1
  KPgain6/1 -> Out6/1
  Output2/1 -> KPgain3/1
  KPgain4/1 -> Out4/1

== system DSR_sim/KPgain2 ==
  Output : Inport
  Output1 : Inport  Port=2
  Output2 : Inport  Port=3
  Output3 : Inport  Port=4
  Output4 : Inport  Port=5
  Output5 : Inport  Port=6
  KPgain{1..6} (6 alike) : Gain  Gain=betac*alpha^2
  Out1 : Outport
  Out2 : Outport  Port=2
  Out3 : Outport  Port=3
  Out4 : Outport  Port=4
  Out5 : Outport  Port=5
  Out6 : Outport  Port=6
  wires:
  Output4/1 -> KPgain5/1
  KPgain1/1 -> Out1/1
  KPgain2/1 -> Out2/1
  KPgain5/1 -> Out5/1
  Output/1 -> KPgain1/1
  Output3/1 -> KPgain4/1
  Output5/1 -> KPgain6/1
  Output1/1 -> KPgain2/1
  KPgain3/1 -> Out3/1
  KPgain6/1 -> Out6/1
  Output2/1 -> KPgain3/1
  KPgain4/1 -> Out4/1

== system DSR_sim/KPgain3 ==
  Output : Inport
  Output1 : Inport  Port=2
  Output2 : Inport  Port=3
  Output3 : Inport  Port=4
  Output4 : Inport  Port=5
  Output5 : Inport  Port=6
  KPgain{1..6} (6 alike) : Gain  Gain=alpha^2
  Out1 : Outport
  Out2 : Outport  Port=2
  Out3 : Outport  Port=3
  Out4 : Outport  Port=4
  Out5 : Outport  Port=5
  Out6 : Outport  Port=6
  wires:
  Output4/1 -> KPgain5/1
  KPgain1/1 -> Out1/1
  KPgain2/1 -> Out2/1
  KPgain5/1 -> Out5/1
  Output/1 -> KPgain1/1
  Output3/1 -> KPgain4/1
  Output5/1 -> KPgain6/1
  Output1/1 -> KPgain2/1
  KPgain3/1 -> Out3/1
  KPgain6/1 -> Out6/1
  Output2/1 -> KPgain3/1
  KPgain4/1 -> Out4/1

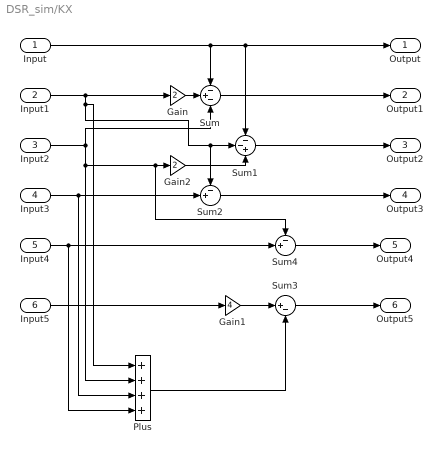
== system DSR_sim/KX ==
  Input : Inport
  Input1 : Inport  Port=2
  Input2 : Inport  Port=3
  Input3 : Inport  Port=4
  Input4 : Inport  Port=5
  Input5 : Inport  Port=6
  Gain : Gain  Gain=2
  Gain1 : Gain  Gain=4
  Gain2 : Gain  Gain=2
  Plus : Sum  Inputs=++++
  Sum : Sum  Inputs=-+-
  Sum1 : Sum  Inputs=--+
  Sum2 : Sum  Inputs=-+|
  Sum3 : Sum  Inputs=|+-
  Sum4 : Sum  Inputs=-+|
  Output : Outport
  Output1 : Outport  Port=2
  Output2 : Outport  Port=3
  Output3 : Outport  Port=4
  Output4 : Outport  Port=5
  Output5 : Outport  Port=6
  wires:
  Input1/1 -> Sum1/2, Sum2/1, Plus/1, Gain/1
  Input/1 -> Sum/1, Output/1, Sum1/1
  Input2/1 -> Sum4/1, Gain2/1, Plus/2, Sum/3
  Sum1/1 -> Output2/1
  Input4/1 -> Sum4/2, Plus/4
  Gain/1 -> Sum/2
  Gain2/1 -> Sum1/3
  Sum/1 -> Output1/1
  Plus/1 -> Sum3/2
  Sum3/1 -> Output5/1
  Input5/1 -> Gain1/1
  Sum4/1 -> Output4/1
  Input3/1 -> Sum2/2, Plus/3
  Sum2/1 -> Output3/1
  Gain1/1 -> Sum3/1

== system DSR_sim/KX1 ==
  Input : Inport
  Input1 : Inport  Port=2
  Input2 : Inport  Port=3
  Input3 : Inport  Port=4
  Input4 : Inport  Port=5
  Input5 : Inport  Port=6
  Gain : Gain  Gain=2
  Gain1 : Gain  Gain=4
  Gain2 : Gain  Gain=2
  Plus : Sum  Inputs=++++
  Sum : Sum  Inputs=-+-
  Sum1 : Sum  Inputs=--+
  Sum2 : Sum  Inputs=-+|
  Sum3 : Sum  Inputs=|+-
  Sum4 : Sum  Inputs=-+|
  Output : Outport
  Output1 : Outport  Port=2
  Output2 : Outport  Port=3
  Output3 : Outport  Port=4
  Output4 : Outport  Port=5
  Output5 : Outport  Port=6
  wires:
  Input1/1 -> Sum1/2, Sum2/1, Plus/1, Gain/1
  Input/1 -> Sum/1, Output/1, Sum1/1
  Input2/1 -> Sum4/1, Gain2/1, Plus/2, Sum/3
  Sum1/1 -> Output2/1
  Input4/1 -> Sum4/2, Plus/4
  Gain/1 -> Sum/2
  Gain2/1 -> Sum1/3
  Sum/1 -> Output1/1
  Plus/1 -> Sum3/2
  Sum3/1 -> Output5/1
  Input5/1 -> Gain1/1
  Sum4/1 -> Output4/1
  Input3/1 -> Sum2/2, Plus/3
  Sum2/1 -> Output3/1
  Gain1/1 -> Sum3/1

== system DSR_sim/KX2 ==
  Input : Inport
  Input1 : Inport  Port=2
  Input2 : Inport  Port=3
  Input3 : Inport  Port=4
  Input4 : Inport  Port=5
  Input5 : Inport  Port=6
  Gain : Gain  Gain=2
  Gain1 : Gain  Gain=4
  Gain2 : Gain  Gain=2
  Plus : Sum  Inputs=++++
  Sum : Sum  Inputs=-+-
  Sum1 : Sum  Inputs=--+
  Sum2 : Sum  Inputs=-+|
  Sum3 : Sum  Inputs=|+-
  Sum4 : Sum  Inputs=-+|
  Output : Outport
  Output1 : Outport  Port=2
  Output2 : Outport  Port=3
  Output3 : Outport  Port=4
  Output4 : Outport  Port=5
  Output5 : Outport  Port=6
  wires:
  Input1/1 -> Sum1/2, Sum2/1, Plus/1, Gain/1
  Input/1 -> Sum/1, Output/1, Sum1/1
  Input2/1 -> Sum4/1, Gain2/1, Plus/2, Sum/3
  Sum1/1 -> Output2/1
  Input4/1 -> Sum4/2, Plus/4
  Gain/1 -> Sum/2
  Gain2/1 -> Sum1/3
  Sum/1 -> Output1/1
  Plus/1 -> Sum3/2
  Sum3/1 -> Output5/1
  Input5/1 -> Gain1/1
  Sum4/1 -> Output4/1
  Input3/1 -> Sum2/2, Plus/3
  Sum2/1 -> Output3/1
  Gain1/1 -> Sum3/1

== system DSR_sim/KX3 ==
  Input : Inport
  Input1 : Inport  Port=2
  Input2 : Inport  Port=3
  Input3 : Inport  Port=4
  Input4 : Inport  Port=5
  Input5 : Inport  Port=6
  Gain : Gain  Gain=2
  Gain1 : Gain  Gain=4
  Gain2 : Gain  Gain=2
  Plus : Sum  Inputs=++++
  Sum : Sum  Inputs=-+-
  Sum1 : Sum  Inputs=--+
  Sum2 : Sum  Inputs=-+|
  Sum3 : Sum  Inputs=|+-
  Sum4 : Sum  Inputs=-+|
  Output : Outport
  Output1 : Outport  Port=2
  Output2 : Outport  Port=3
  Output3 : Outport  Port=4
  Output4 : Outport  Port=5
  Output5 : Outport  Port=6
  wires:
  Input1/1 -> Sum1/2, Sum2/1, Plus/1, Gain/1
  Input/1 -> Sum/1, Output/1, Sum1/1
  Input2/1 -> Sum4/1, Gain2/1, Plus/2, Sum/3
  Sum1/1 -> Output2/1
  Input4/1 -> Sum4/2, Plus/4
  Gain/1 -> Sum/2
  Gain2/1 -> Sum1/3
  Sum/1 -> Output1/1
  Plus/1 -> Sum3/2
  Sum3/1 -> Output5/1
  Input5/1 -> Gain1/1
  Sum4/1 -> Output4/1
  Input3/1 -> Sum2/2, Plus/3
  Sum2/1 -> Output3/1
  Gain1/1 -> Sum3/1

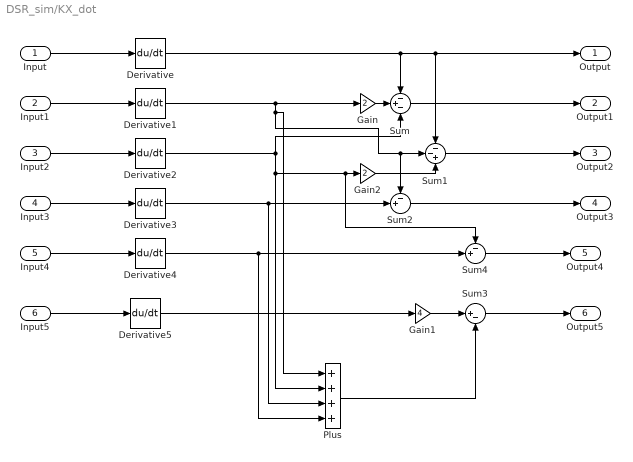
== system DSR_sim/KX_dot ==
  Input : Inport
  Input1 : Inport  Port=2
  Input2 : Inport  Port=3
  Input3 : Inport  Port=4
  Input4 : Inport  Port=5
  Input5 : Inport  Port=6
  Derivative{,1..5} (6 alike) : Derivative
  Gain : Gain  Gain=2
  Gain1 : Gain  Gain=4
  Gain2 : Gain  Gain=2
  Plus : Sum  Inputs=++++
  Sum : Sum  Inputs=-+-
  Sum1 : Sum  Inputs=--+
  Sum2 : Sum  Inputs=-+|
  Sum3 : Sum  Inputs=|+-
  Sum4 : Sum  Inputs=-+|
  Output : Outport
  Output1 : Outport  Port=2
  Output2 : Outport  Port=3
  Output3 : Outport  Port=4
  Output4 : Outport  Port=5
  Output5 : Outport  Port=6
  wires:
  Input1/1 -> Derivative1/1
  Input/1 -> Derivative/1
  Input2/1 -> Derivative2/1
  Sum1/1 -> Output2/1
  Input4/1 -> Derivative4/1
  Gain/1 -> Sum/2
  Gain2/1 -> Sum1/3
  Sum/1 -> Output1/1
  Plus/1 -> Sum3/2
  Sum3/1 -> Output5/1
  Input5/1 -> Derivative5/1
  Sum4/1 -> Output4/1
  Input3/1 -> Derivative3/1
  Sum2/1 -> Output3/1
  Gain1/1 -> Sum3/1
  Derivative/1 -> Sum/1, Output/1, Sum1/1
  Derivative1/1 -> Sum1/2, Sum2/1, Plus/1, Gain/1
  Derivative2/1 -> Sum4/1, Gain2/1, Plus/2, Sum/3
  Derivative3/1 -> Sum2/2, Plus/3
  Derivative4/1 -> Sum4/2, Plus/4
  Derivative5/1 -> Gain1/1

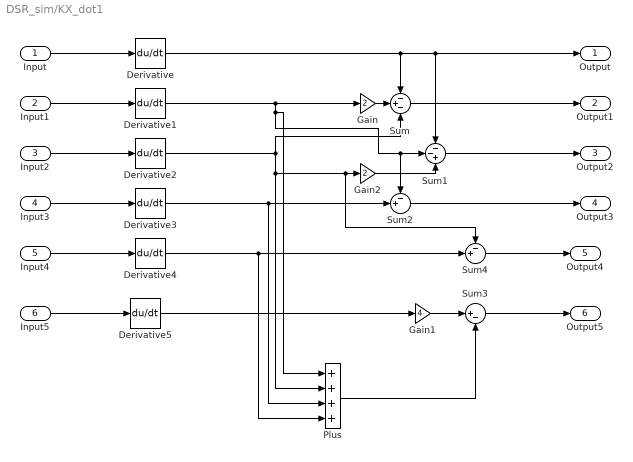
== system DSR_sim/KX_dot1 ==
  Input : Inport
  Input1 : Inport  Port=2
  Input2 : Inport  Port=3
  Input3 : Inport  Port=4
  Input4 : Inport  Port=5
  Input5 : Inport  Port=6
  Derivative{,1..5} (6 alike) : Derivative
  Gain : Gain  Gain=2
  Gain1 : Gain  Gain=4
  Gain2 : Gain  Gain=2
  Plus : Sum  Inputs=++++
  Sum : Sum  Inputs=-+-
  Sum1 : Sum  Inputs=--+
  Sum2 : Sum  Inputs=-+|
  Sum3 : Sum  Inputs=|+-
  Sum4 : Sum  Inputs=-+|
  Output : Outport
  Output1 : Outport  Port=2
  Output2 : Outport  Port=3
  Output3 : Outport  Port=4
  Output4 : Outport  Port=5
  Output5 : Outport  Port=6
  wires:
  Input1/1 -> Derivative1/1
  Input/1 -> Derivative/1
  Input2/1 -> Derivative2/1
  Sum1/1 -> Output2/1
  Input4/1 -> Derivative4/1
  Gain/1 -> Sum/2
  Gain2/1 -> Sum1/3
  Sum/1 -> Output1/1
  Plus/1 -> Sum3/2
  Sum3/1 -> Output5/1
  Input5/1 -> Derivative5/1
  Sum4/1 -> Output4/1
  Input3/1 -> Derivative3/1
  Sum2/1 -> Output3/1
  Gain1/1 -> Sum3/1
  Derivative/1 -> Sum/1, Output/1, Sum1/1
  Derivative1/1 -> Sum1/2, Sum2/1, Plus/1, Gain/1
  Derivative2/1 -> Sum4/1, Gain2/1, Plus/2, Sum/3
  Derivative3/1 -> Sum2/2, Plus/3
  Derivative4/1 -> Sum4/2, Plus/4
  Derivative5/1 -> Gain1/1

== system DSR_sim/KX_dot2 ==
  Input : Inport
  Input1 : Inport  Port=2
  Input2 : Inport  Port=3
  Input3 : Inport  Port=4
  Input4 : Inport  Port=5
  Input5 : Inport  Port=6
  Gain : Gain  Gain=2
  Gain1 : Gain  Gain=4
  Gain2 : Gain  Gain=2
  Plus : Sum  Inputs=++++
  Sum : Sum  Inputs=-+-
  Sum1 : Sum  Inputs=--+
  Sum2 : Sum  Inputs=-+|
  Sum3 : Sum  Inputs=|+-
  Sum4 : Sum  Inputs=-+|
  Output : Outport
  Output1 : Outport  Port=2
  Output2 : Outport  Port=3
  Output3 : Outport  Port=4
  Output4 : Outport  Port=5
  Output5 : Outport  Port=6
  wires:
  Sum1/1 -> Output2/1
  Gain/1 -> Sum/2
  Gain2/1 -> Sum1/3
  Sum/1 -> Output1/1
  Plus/1 -> Sum3/2
  Sum3/1 -> Output5/1
  Sum4/1 -> Output4/1
  Sum2/1 -> Output3/1
  Gain1/1 -> Sum3/1
  Input/1 -> Sum/1, Output/1, Sum1/1
  Input1/1 -> Sum1/2, Sum2/1, Plus/1, Gain/1
  Input2/1 -> Sum4/1, Gain2/1, Plus/2, Sum/3
  Input3/1 -> Sum2/2, Plus/3
  Input4/1 -> Sum4/2, Plus/4
  Input5/1 -> Gain1/1

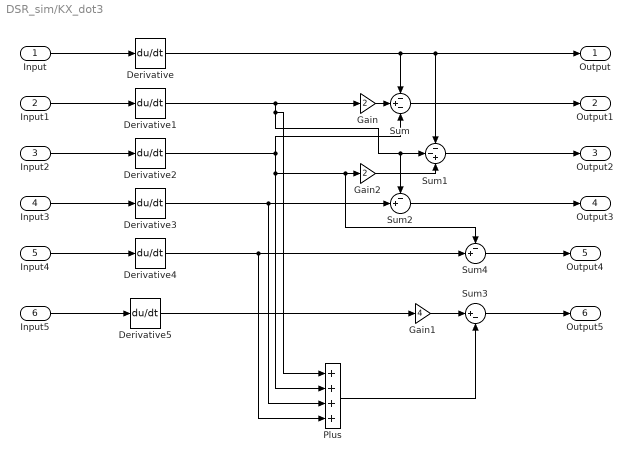
== system DSR_sim/KX_dot3 ==
  Input : Inport
  Input1 : Inport  Port=2
  Input2 : Inport  Port=3
  Input3 : Inport  Port=4
  Input4 : Inport  Port=5
  Input5 : Inport  Port=6
  Derivative{,1..5} (6 alike) : Derivative
  Gain : Gain  Gain=2
  Gain1 : Gain  Gain=4
  Gain2 : Gain  Gain=2
  Plus : Sum  Inputs=++++
  Sum : Sum  Inputs=-+-
  Sum1 : Sum  Inputs=--+
  Sum2 : Sum  Inputs=-+|
  Sum3 : Sum  Inputs=|+-
  Sum4 : Sum  Inputs=-+|
  Output : Outport
  Output1 : Outport  Port=2
  Output2 : Outport  Port=3
  Output3 : Outport  Port=4
  Output4 : Outport  Port=5
  Output5 : Outport  Port=6
  wires:
  Input1/1 -> Derivative1/1
  Input/1 -> Derivative/1
  Input2/1 -> Derivative2/1
  Sum1/1 -> Output2/1
  Input4/1 -> Derivative4/1
  Gain/1 -> Sum/2
  Gain2/1 -> Sum1/3
  Sum/1 -> Output1/1
  Plus/1 -> Sum3/2
  Sum3/1 -> Output5/1
  Input5/1 -> Derivative5/1
  Sum4/1 -> Output4/1
  Input3/1 -> Derivative3/1
  Sum2/1 -> Output3/1
  Gain1/1 -> Sum3/1
  Derivative/1 -> Sum/1, Output/1, Sum1/1
  Derivative1/1 -> Sum1/2, Sum2/1, Plus/1, Gain/1
  Derivative2/1 -> Sum4/1, Gain2/1, Plus/2, Sum/3
  Derivative3/1 -> Sum2/2, Plus/3
  Derivative4/1 -> Sum4/2, Plus/4
  Derivative5/1 -> Gain1/1

== system DSR_sim/system ==
  In1 : Inport
  In2 : Inport  Port=2
  In3 : Inport  Port=3
  In4 : Inport  Port=4
  In5 : Inport  Port=5
  In6 : Inport  Port=6
  Transfer Fcn{,1..5} (6 alike) : TransferFcn  Denominator=[1 0 0]
  Ag1 : Outport
  Ag2 : Outport  Port=2
  Ag3 : Outport  Port=3
  Ag4 : Outport  Port=4
  Ag5 : Outport  Port=5
  Ag6 : Outport  Port=6
  wires:
  Transfer Fcn4/1 -> Ag5/1
  In1/1 -> Transfer Fcn/1
  Transfer Fcn/1 -> Ag1/1
  In3/1 -> Transfer Fcn2/1
  Transfer Fcn2/1 -> Ag3/1
  In2/1 -> Transfer Fcn1/1
  In5/1 -> Transfer Fcn4/1
  Transfer Fcn1/1 -> Ag2/1
  In6/1 -> Transfer Fcn5/1
  In4/1 -> Transfer Fcn3/1
  Transfer Fcn5/1 -> Ag6/1
  Transfer Fcn3/1 -> Ag4/1

== system DSR_sim/system1 ==
  In1 : Inport
  In2 : Inport  Port=2
  In3 : Inport  Port=3
  In4 : Inport  Port=4
  In5 : Inport  Port=5
  In6 : Inport  Port=6
  Transfer Fcn{,1..5} (6 alike) : TransferFcn  Denominator=[1 0 0]
  Ag1 : Outport
  Ag2 : Outport  Port=2
  Ag3 : Outport  Port=3
  Ag4 : Outport  Port=4
  Ag5 : Outport  Port=5
  Ag6 : Outport  Port=6
  wires:
  Transfer Fcn4/1 -> Ag5/1
  In1/1 -> Transfer Fcn/1
  Transfer Fcn/1 -> Ag1/1
  In3/1 -> Transfer Fcn2/1
  Transfer Fcn2/1 -> Ag3/1
  In2/1 -> Transfer Fcn1/1
  In5/1 -> Transfer Fcn4/1
  Transfer Fcn1/1 -> Ag2/1
  In6/1 -> Transfer Fcn5/1
  In4/1 -> Transfer Fcn3/1
  Transfer Fcn5/1 -> Ag6/1
  Transfer Fcn3/1 -> Ag4/1

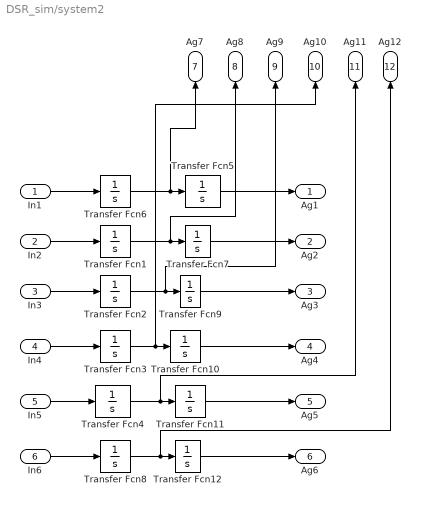
== system DSR_sim/system2 ==
  In1 : Inport
  In2 : Inport  Port=2
  In3 : Inport  Port=3
  In4 : Inport  Port=4
  In5 : Inport  Port=5
  In6 : Inport  Port=6
  Transfer Fcn{1..12} (12 alike) : TransferFcn  Denominator=[1 0]
  Ag1 : Outport
  Ag2 : Outport  Port=2
  Ag3 : Outport  Port=3
  Ag4 : Outport  Port=4
  Ag5 : Outport  Port=5
  Ag6 : Outport  Port=6
  Ag7 : Outport  Port=7
  Ag8 : Outport  Port=8
  Ag9 : Outport  Port=9
  Ag10 : Outport  Port=10
  Ag11 : Outport  Port=11
  Ag12 : Outport  Port=12
  wires:
  Transfer Fcn11/1 -> Ag5/1
  In1/1 -> Transfer Fcn6/1
  Transfer Fcn5/1 -> Ag1/1
  In3/1 -> Transfer Fcn2/1
  Transfer Fcn9/1 -> Ag3/1
  In2/1 -> Transfer Fcn1/1
  In5/1 -> Transfer Fcn4/1
  Transfer Fcn7/1 -> Ag2/1
  In6/1 -> Transfer Fcn8/1
  In4/1 -> Transfer Fcn3/1
  Transfer Fcn12/1 -> Ag6/1
  Transfer Fcn10/1 -> Ag4/1
  Transfer Fcn6/1 -> Ag7/1, Transfer Fcn5/1
  Transfer Fcn1/1 -> Ag8/1, Transfer Fcn7/1
  Transfer Fcn2/1 -> Ag9/1, Transfer Fcn9/1
  Transfer Fcn3/1 -> Ag10/1, Transfer Fcn10/1
  Transfer Fcn4/1 -> Ag11/1, Transfer Fcn11/1
  Transfer Fcn8/1 -> Ag12/1, Transfer Fcn12/1

== system DSR_sim/DerEst/Derivative Estimator ==
  pos : Inport
  DSRdelay : Subsystem
  LPF : TransferFcn  Numerator=[omega^2]  Denominator=[delay^2 2*omega*delay^2 omega^2*delay^2]
  est : Outport
  wires:
  LPF/1 -> DSRdelay/1(Input)
  DSRdelay/1(Out1) -> est/1
  pos/1 -> LPF/1

== system DSR_sim/DerEst/Derivative Estimator1 ==
  pos : Inport
  DSRdelay : Subsystem
  LPF : TransferFcn  Numerator=[omega^2]  Denominator=[delay^2 2*omega*delay^2 omega^2*delay^2]
  est : Outport
  wires:
  LPF/1 -> DSRdelay/1(Input)
  DSRdelay/1(Out1) -> est/1
  pos/1 -> LPF/1

== system DSR_sim/DerEst/Derivative Estimator2 ==
  pos : Inport
  DSRdelay : Subsystem
  LPF : TransferFcn  Numerator=[omega^2]  Denominator=[delay^2 2*omega*delay^2 omega^2*delay^2]
  est : Outport
  wires:
  LPF/1 -> DSRdelay/1(Input)
  DSRdelay/1(Out1) -> est/1
  pos/1 -> LPF/1

== system DSR_sim/DerEst/Derivative Estimator3 ==
  pos : Inport
  DSRdelay : Subsystem
  LPF : TransferFcn  Numerator=[omega^2]  Denominator=[delay^2 2*omega*delay^2 omega^2*delay^2]
  est : Outport
  wires:
  LPF/1 -> DSRdelay/1(Input)
  DSRdelay/1(Out1) -> est/1
  pos/1 -> LPF/1

== system DSR_sim/DerEst/Derivative Estimator4 ==
  pos : Inport
  DSRdelay : Subsystem
  LPF : TransferFcn  Numerator=[omega^2]  Denominator=[delay^2 2*omega*delay^2 omega^2*delay^2]
  est : Outport
  wires:
  LPF/1 -> DSRdelay/1(Input)
  DSRdelay/1(Out1) -> est/1
  pos/1 -> LPF/1

== system DSR_sim/DerEst/Derivative Estimator5 ==
  pos : Inport
  DSRdelay : Subsystem
  LPF : TransferFcn  Numerator=[omega^2]  Denominator=[delay^2 2*omega*delay^2 omega^2*delay^2]
  est : Outport
  wires:
  LPF/1 -> DSRdelay/1(Input)
  DSRdelay/1(Out1) -> est/1
  pos/1 -> LPF/1

== system DSR_sim/DerEst1/Derivative Estimator ==
  pos : Inport
  DSRdelay : Subsystem
  LPF : TransferFcn  Numerator=[omega^2]  Denominator=[delay^2 2*omega*delay^2 omega^2*delay^2]
  est : Outport
  wires:
  LPF/1 -> DSRdelay/1(Input)
  DSRdelay/1(Out1) -> est/1
  pos/1 -> LPF/1

== system DSR_sim/DerEst1/Derivative Estimator1 ==
  pos : Inport
  DSRdelay : Subsystem
  LPF : TransferFcn  Numerator=[omega^2]  Denominator=[delay^2 2*omega*delay^2 omega^2*delay^2]
  est : Outport
  wires:
  LPF/1 -> DSRdelay/1(Input)
  DSRdelay/1(Out1) -> est/1
  pos/1 -> LPF/1

== system DSR_sim/DerEst1/Derivative Estimator2 ==
  pos : Inport
  DSRdelay : Subsystem
  LPF : TransferFcn  Numerator=[omega^2]  Denominator=[delay^2 2*omega*delay^2 omega^2*delay^2]
  est : Outport
  wires:
  LPF/1 -> DSRdelay/1(Input)
  DSRdelay/1(Out1) -> est/1
  pos/1 -> LPF/1

== system DSR_sim/DerEst1/Derivative Estimator3 ==
  pos : Inport
  DSRdelay : Subsystem
  LPF : TransferFcn  Numerator=[omega^2]  Denominator=[delay^2 2*omega*delay^2 omega^2*delay^2]
  est : Outport
  wires:
  LPF/1 -> DSRdelay/1(Input)
  DSRdelay/1(Out1) -> est/1
  pos/1 -> LPF/1

== system DSR_sim/DerEst1/Derivative Estimator4 ==
  pos : Inport
  DSRdelay : Subsystem
  LPF : TransferFcn  Numerator=[omega^2]  Denominator=[delay^2 2*omega*delay^2 omega^2*delay^2]
  est : Outport
  wires:
  LPF/1 -> DSRdelay/1(Input)
  DSRdelay/1(Out1) -> est/1
  pos/1 -> LPF/1

== system DSR_sim/DerEst1/Derivative Estimator5 ==
  pos : Inport
  DSRdelay : Subsystem
  LPF : TransferFcn  Numerator=[omega^2]  Denominator=[delay^2 2*omega*delay^2 omega^2*delay^2]
  est : Outport
  wires:
  LPF/1 -> DSRdelay/1(Input)
  DSRdelay/1(Out1) -> est/1
  pos/1 -> LPF/1

== system DSR_sim/DerEst2/Derivative Estimator ==
  pos : Inport
  DSRdelay : Subsystem
  LPF : TransferFcn  Numerator=[omega^2]  Denominator=[delay^2 2*omega*delay^2 omega^2*delay^2]
  est : Outport
  wires:
  LPF/1 -> DSRdelay/1(Input)
  DSRdelay/1(Out1) -> est/1
  pos/1 -> LPF/1

== system DSR_sim/DerEst2/Derivative Estimator1 ==
  pos : Inport
  DSRdelay : Subsystem
  LPF : TransferFcn  Numerator=[omega^2]  Denominator=[delay^2 2*omega*delay^2 omega^2*delay^2]
  est : Outport
  wires:
  LPF/1 -> DSRdelay/1(Input)
  DSRdelay/1(Out1) -> est/1
  pos/1 -> LPF/1

== system DSR_sim/DerEst2/Derivative Estimator2 ==
  pos : Inport
  DSRdelay : Subsystem
  LPF : TransferFcn  Numerator=[omega^2]  Denominator=[delay^2 2*omega*delay^2 omega^2*delay^2]
  est : Outport
  wires:
  LPF/1 -> DSRdelay/1(Input)
  DSRdelay/1(Out1) -> est/1
  pos/1 -> LPF/1

== system DSR_sim/DerEst2/Derivative Estimator3 ==
  pos : Inport
  DSRdelay : Subsystem
  LPF : TransferFcn  Numerator=[omega^2]  Denominator=[delay^2 2*omega*delay^2 omega^2*delay^2]
  est : Outport
  wires:
  LPF/1 -> DSRdelay/1(Input)
  DSRdelay/1(Out1) -> est/1
  pos/1 -> LPF/1

== system DSR_sim/DerEst2/Derivative Estimator4 ==
  pos : Inport
  DSRdelay : Subsystem
  LPF : TransferFcn  Numerator=[omega^2]  Denominator=[delay^2 2*omega*delay^2 omega^2*delay^2]
  est : Outport
  wires:
  LPF/1 -> DSRdelay/1(Input)
  DSRdelay/1(Out1) -> est/1
  pos/1 -> LPF/1

== system DSR_sim/DerEst2/Derivative Estimator5 ==
  pos : Inport
  DSRdelay : Subsystem
  LPF : TransferFcn  Numerator=[omega^2]  Denominator=[delay^2 2*omega*delay^2 omega^2*delay^2]
  est : Outport
  wires:
  LPF/1 -> DSRdelay/1(Input)
  DSRdelay/1(Out1) -> est/1
  pos/1 -> LPF/1

== system DSR_sim/DerEst/Derivative Estimator/DSRdelay ==
  Input : Inport
  Gain : Gain  Gain=2
  Sum : Sum  Inputs=-++
  Transport Delay1 : TransportDelay  DelayTime=2*delay
  Transport Delay2 : TransportDelay  DelayTime=delay
  Out1 : Outport
  wires:
  Input/1 -> Transport Delay2/1, Transport Delay1/1, Sum/2
  Transport Delay2/1 -> Gain/1
  Transport Delay1/1 -> Sum/3
  Gain/1 -> Sum/1
  Sum/1 -> Out1/1

== system DSR_sim/DerEst/Derivative Estimator1/DSRdelay ==
  Input : Inport
  Gain : Gain  Gain=2
  Sum : Sum  Inputs=-++
  Transport Delay1 : TransportDelay  DelayTime=2*delay
  Transport Delay2 : TransportDelay  DelayTime=delay
  Out1 : Outport
  wires:
  Input/1 -> Transport Delay2/1, Transport Delay1/1, Sum/2
  Transport Delay2/1 -> Gain/1
  Transport Delay1/1 -> Sum/3
  Gain/1 -> Sum/1
  Sum/1 -> Out1/1
